simulink model "ofdm_14b"  (Simulink 8.5)
settings: Solver=FixedStepDiscrete  SolverMode=SingleTasking  StartTime=0.0  StopTime=inf  MaxStep=1/(100*40e6)  RelTol=1e-3
PreLoadFcn:
  | Fsymbol              = .5e6;         % Symbol rate
  | D=8;  % decimation / interpolation
  | Bits_per_Symbol = 2;
  | Fbit  = Bits_per_Symbol*Fsymbol;
  | 
  | FFT_Size  = 64;
  | Cyclic        = 16;
  | Pilots         = 16;
  | Pilot_Level = 8;
  | Zero_Pad  = 3;
  | QAM_Level = 6;
  | 
  | OFDM_Frame =  FFT_Size+Cyclic;
  | Symbols_per_Frame = FFT_Size-Pilots-Zero_Pad;
  | 
  | Bits_per_Frame = Bits_per_Symbol*Symbols_per_Frame;
  | 
  | F_nco = Fsymbol*D*OFDM_Frame/(Symbols_per_Frame);
  | nco_nominal=2/D;
  | 
  | 
  | Fdelay = 8;  % rrc filter delay
  | Alpha = .25;  % excess BW
  | %rrc_coef=rcosine(1,D,'fir/sqrt',Alpha,Fdelay);
  | %rrc_coef=rrc_coef/sum(rrc_coef);
  | 
  | DPS=fdesign.pulseshaping(D,'Square Root Raised Cosine','Nsym,Beta',2*Fdelay,Alpha);
  | Hd=design(DPS);
  | rrc_coef=Hd.Numerator;
  | % force DC gain to unity.
  | rrc_coef=rrc_coef/sum(rrc_coef);
  | 
  | % coefficents for Farrow filter
  | b3 = [1/6 -1/2  1/2 -1/6];
  | b2 = [1/2 -1    1/2  0];
  | b1 = [1/3  1/2 -1    1/6];
  | b0 = [0    1    0    0];
StartFcn:
  | tic
StopFcn:
  | trun=toc
undefined symbols (not defined in the file): dfilt, Fs, j, magnitude
libraries: simulink x16, dspobslib x5, dspxfrm3 x4, dspstat3 x4, dspsnks4 x3, commchan3 x2, commrandsrc2 x2, commdigbbndam3 x2, dspsrcs4 x2, dspbuff3 x2, dsppolyfun x1, commsink2 x1
(part 2 of 2)

== system ofdm_14b/OFDM Transmitter with Variable Symbol Timing and Carrier Frequency Error/OFDM Symbol Gen/OFDM Generator ==
  note: set data signal level
  in_data : Inport  OutDataTypeStr=uint8
  Enable : EnablePort
  Buffer : Buffer  N=Bits_per_Frame  TreatMby1Signals=One channel
  Frame Conversion : FrameConversion  OutFrame=Sample-based
  Gain : Gain  Gain=D
  Gain1 : Gain  Gain=QAM_Level  SaturateOnIntegerOverflow=on  OutDataTypeStr=Inherit: Same as input  ParamDataTypeStr=Inherit: Same as input
  OFDM Transmitter1 : Subsystem
      mask Display: disp('OFDM\nTransmitter')
  Rectangular QAM Modulator Baseband1 : commdigbbndam3/Rectangular QAM Modulator Baseband  M=4  InType=Bit  Enc=Binary  Mapping=[0:15]  PowType=Min. distance between symbols  MinDist=2  AvgPow=1  PeakPow=1  Ph=0  outDtype=Fixed-point  outWordLen=12  outUDDataType=sfix(16)  outFracLenMode=User-defined  outFracLen=7
  Out1 : Outport
  wires:
  Buffer/1 -> Rectangular QAM Modulator Baseband1/1
  OFDM Transmitter1/1(Out) -> Gain/1
  Rectangular QAM Modulator Baseband1/1 -> Gain1/1
  Gain/1 -> Frame Conversion/1
  Gain1/1 -> OFDM Transmitter1/1(In)
  Frame Conversion/1 -> Out1/1
  in_data/1 -> Buffer/1

== system ofdm_14b/OFDM Transmitter with Variable Symbol Timing and Carrier Frequency Error/Timing Control Unit1/S&H 1 ==
  In1 : Inport
  Enable : EnablePort
  Out1 : Outport
  wires:
  In1/1 -> Out1/1

== system ofdm_14b/OFDM Transmitter with Variable Symbol Timing and Carrier Frequency Error/Timing Control Unit1/Scaling1 ==
  note: This Division can be eliminated
      | and replaced by a mpy by constant
      | for small variations (< 1%)
      | about an operating point.
  In1 : Inport
  In2 : Inport  Port=2
  Add : Sum  Inputs=-+
  Constant : Constant
  Divide : Product  Inputs=*/
  Out1 : Outport
  wires:
  In2/1 -> Divide/2
  In1/1 -> Add/1
  Constant/1 -> Add/2
  Add/1 -> Divide/1
  Divide/1 -> Out1/1

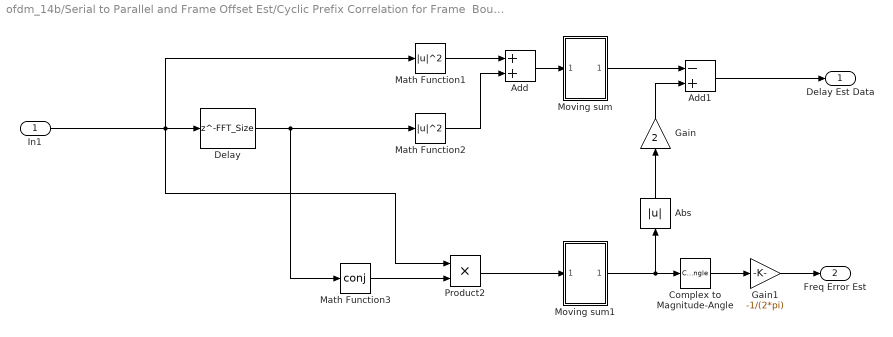
== system ofdm_14b/Serial to Parallel and Frame Offset Est/Cyclic Prefix Correlation for Frame  Boundary Estimation/Estimators ==
  In1 : Inport
  Abs : Abs
  Add : Sum
  Add1 : Sum  Inputs=-+
  Complex to Magnitude-Angle : ComplexToMagnitudeAngle  Output=Angle
  Delay : Delay  DelayLength=FFT_Size  InitialCondition=0
  Gain : Gain  Gain=2
  Gain1 : Gain  Gain=-1/(2*pi)
  Math Function1 : Math  Operator=magnitude^2  SaturateOnIntegerOverflow=on
  Math Function2 : Math  Operator=magnitude^2  SaturateOnIntegerOverflow=on
  Math Function3 : Math  Operator=conj  SaturateOnIntegerOverflow=on
  Moving sum : Subsystem
  Moving sum1 : Subsystem
  Product2 : Product  RndMeth=Zero
  Delay Est Data : Outport
  Freq Error Est : Outport  Port=2
  wires:
  In1/1 -> Product2/1, Delay/1, Math Function1/1
  Gain1/1 -> Freq Error Est/1
  Complex to Magnitude-Angle/1 -> Gain1/1
  Math Function3/1 -> Product2/2
  Gain/1 -> Add1/2
  Abs/1 -> Gain/1
  Add1/1 -> Delay Est Data/1
  Moving sum/1(Out1) -> Add1/1
  Moving sum1/1(Out1) -> Complex to Magnitude-Angle/1, Abs/1
  Product2/1 -> Moving sum1/1(In1)
  Add/1 -> Moving sum/1(In1)
  Math Function2/1 -> Add/2
  Math Function1/1 -> Add/1
  Delay/1 -> Math Function3/1, Math Function2/1

== system ofdm_14b/Serial to Parallel and Frame Offset Est/Cyclic Prefix Correlation for Frame  Boundary Estimation/Find max ==
  In1 : Inport
  Enable : EnablePort
  Add : Sum  Inputs=+-
  Constant : Constant  Value=OFDM_Frame/2
  Frame Conversion : FrameConversion  OutFrame=Sample-based
  Maximum : dspstat3/Maximum  fcn=Index  reset=None  InputProcessing=Columns as channels (frame based)  indexBase=One  operateOver=Each column  Dimension=1  colComp=on  operation=maximum  roiEnable=off  roiType=Rectangles  roiPortion=Entire ROI  roiOutput=Individual statistics for each ROI  roiFlag=off  accumDataTypeStr=Inherit: Same as product output  accumLastDataTypeStr=Inherit: Same as product output  roundingMode=Floor  overflowMode=off
  Moving sum : Subsystem
  reorder to center 0 point : Selector  InputPortWidth=80  Indices=[(OFDM_Frame/2+1):80 1:OFDM_Frame/2]
  Frame Offset Est : Outport  InitialOutput=0
  wires:
  In1/1 -> reorder to center 0 point/1
  Maximum/1 -> Frame Conversion/1
  reorder to center 0 point/1 -> Maximum/1
  Frame Conversion/1 -> Add/1
  Add/1 -> Moving sum/1(In1)
  Constant/1 -> Add/2
  Moving sum/1(Out1) -> Frame Offset Est/1

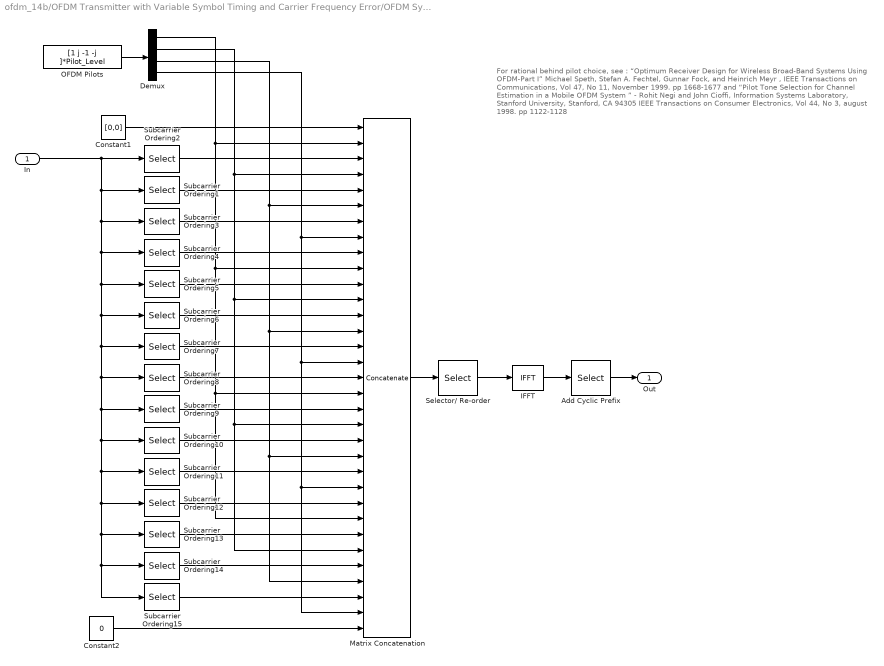
== system ofdm_14b/OFDM Transmitter with Variable Symbol Timing and Carrier Frequency Error/OFDM Symbol Gen/OFDM Generator/OFDM Transmitter1 ==
  note: For rational behind pilot choice, see :
      | “Optimum Receiver Design for Wireless Broad-Band Systems Using OFDM-Part I”
      | Michael Speth, Stefan A. Fechtel, Gunnar Fock, and Heinrich Meyr ,
      |  IEEE Transactions on Communications, Vol 47, No 11, November 1999. pp 1668-1677
      | and
      | “Pilot Tone Selection for Channel Estimation in a Mobile OFDM System ” -
      |  Rohit Negi and John Cioffi, Information Systems Laboratory, Stanford University, Stanford, CA 94305
      | IEEE Transactions on Consumer Electronics, Vol 44, No 3, august 1998. pp 1122-1128
  In : Inport
  Add Cyclic Prefix : Selector  InputPortWidth=64  Indices=[49:64 1:64]
  Constant1 : Constant  Value=[0,0]  OutDataTypeStr=fixdt(1,12,7)
  Constant2 : Constant  Value=0  OutDataTypeStr=fixdt(1,12,7)
  Demux : Demux
  IFFT : dspxfrm3/IFFT  CompMethod=Table lookup  TableOpt=HYBRID  TableOptActive=Speed  BitRevOrder=off  cs_in=off  SkipNorm=on  InheritFFTLength=on  FFTLength=64  WrapInput=on  mode=Complex  outSamplingMode=Frame based  RowConvenienceOn=on  FFTImplementation=Auto  firstCoeffDataTypeStr=Inherit: Same word length as input  firstCoeffLastDataTypeStr=Inherit: Same word length as input  outputMin=[]  outputMax=[]  roundingMode=Floor  overflowMode=off
  Matrix Concatenation : Concatenate  NumInputs=33  Mode=Multidimensional array
  OFDM Pilots : Constant  Value="[1 j -1 -j   ]*Pilot_Level"  OutDataTypeStr=fixdt(1,12,7)
  Selector/ Re-order : Selector  InputPortWidth=64  Indices=[33:64 1:32]
  Subcarrier Ordering1 : Selector  InputPortWidth=Symbols_per_Frame  Indices=4:6
  Subcarrier Ordering10 : Selector  InputPortWidth=Symbols_per_Frame  Indices=28:30
  Subcarrier Ordering11 : Selector  InputPortWidth=Symbols_per_Frame  Indices=31:33
  Subcarrier Ordering12 : Selector  InputPortWidth=Symbols_per_Frame  Indices=34:36
  Subcarrier Ordering13 : Selector  InputPortWidth=Symbols_per_Frame  Indices=37:39
  Subcarrier Ordering14 : Selector  InputPortWidth=Symbols_per_Frame  Indices=40:42
  Subcarrier Ordering15 : Selector  InputPortWidth=Symbols_per_Frame  Indices=43:45
  Subcarrier Ordering2 : Selector  InputPortWidth=Symbols_per_Frame  Indices=1:3
  Subcarrier Ordering3 : Selector  InputPortWidth=Symbols_per_Frame  Indices=7:9
  Subcarrier Ordering4 : Selector  InputPortWidth=Symbols_per_Frame  Indices=10:12
  Subcarrier Ordering5 : Selector  InputPortWidth=Symbols_per_Frame  Indices=13:15
  Subcarrier Ordering6 : Selector  InputPortWidth=Symbols_per_Frame  Indices=16:18
  Subcarrier Ordering7 : Selector  InputPortWidth=Symbols_per_Frame  Indices=19:21
  Subcarrier Ordering8 : Selector  InputPortWidth=Symbols_per_Frame  Indices=22:24
  Subcarrier Ordering9 : Selector  InputPortWidth=Symbols_per_Frame  Indices=25:27
  Out : Outport
  wires:
  In/1 -> Subcarrier Ordering14/1, Subcarrier Ordering15/1, Subcarrier Ordering13/1, Subcarrier Ordering12/1, Subcarrier Ordering11/1, Subcarrier Ordering10/1, Subcarrier Ordering9/1, Subcarrier Ordering8/1, Subcarrier Ordering7/1, Subcarrier Ordering6/1, Subcarrier Ordering5/1, Subcarrier Ordering4/1, Subcarrier Ordering3/1, Subcarrier Ordering1/1, Subcarrier Ordering2/1
  IFFT/1 -> Add Cyclic Prefix/1
  Matrix Concatenation/1 -> Selector/ Re-order/1
  Selector/ Re-order/1 -> IFFT/1
  Subcarrier Ordering2/1 -> Matrix Concatenation/3
  Subcarrier Ordering1/1 -> Matrix Concatenation/5
  Subcarrier Ordering3/1 -> Matrix Concatenation/7
  Subcarrier Ordering4/1 -> Matrix Concatenation/9
  Subcarrier Ordering5/1 -> Matrix Concatenation/11
  Subcarrier Ordering6/1 -> Matrix Concatenation/13
  Subcarrier Ordering7/1 -> Matrix Concatenation/15
  Subcarrier Ordering8/1 -> Matrix Concatenation/17
  Subcarrier Ordering9/1 -> Matrix Concatenation/19
  Subcarrier Ordering10/1 -> Matrix Concatenation/21
  Subcarrier Ordering11/1 -> Matrix Concatenation/23
  Subcarrier Ordering12/1 -> Matrix Concatenation/25
  Subcarrier Ordering13/1 -> Matrix Concatenation/27
  Subcarrier Ordering14/1 -> Matrix Concatenation/29
  Subcarrier Ordering15/1 -> Matrix Concatenation/31
  Add Cyclic Prefix/1 -> Out/1
  Constant1/1 -> Matrix Concatenation/1
  Constant2/1 -> Matrix Concatenation/33
  Demux/2 -> Matrix Concatenation/4, Matrix Concatenation/12, Matrix Concatenation/20, Matrix Concatenation/28
  Demux/3 -> Matrix Concatenation/6, Matrix Concatenation/14, Matrix Concatenation/22, Matrix Concatenation/30
  Demux/4 -> Matrix Concatenation/8, Matrix Concatenation/16, Matrix Concatenation/24, Matrix Concatenation/32
  OFDM Pilots/1 -> Demux/1
  Demux/1 -> Matrix Concatenation/26, Matrix Concatenation/18, Matrix Concatenation/10, Matrix Concatenation/2

== system ofdm_14b/Serial to Parallel and Frame Offset Est/Cyclic Prefix Correlation for Frame  Boundary Estimation/Estimators/Moving sum ==
  In1 : Inport
  Gain : Gain  Gain=1/Cyclic  SaturateOnIntegerOverflow=on  OutDataTypeStr=Inherit: Same as input  ParamDataTypeStr=Inherit: Same as input
  Integer Delay : Delay  DelayLength=Cyclic  InputProcessing=Inherited
  Integer Delay1 : Delay  DelayLength=1  InputProcessing=Inherited
  Sum2 : Sum  Inputs=|+-
  Sum3 : Sum  Inputs=|++
  Out1 : Outport
  wires:
  Gain/1 -> Out1/1
  In1/1 -> Sum2/1, Integer Delay/1
  Sum2/1 -> Sum3/1
  Integer Delay1/1 -> Sum3/2
  Sum3/1 -> Gain/1, Integer Delay1/1
  Integer Delay/1 -> Sum2/2

== system ofdm_14b/Serial to Parallel and Frame Offset Est/Cyclic Prefix Correlation for Frame  Boundary Estimation/Estimators/Moving sum1 ==
  In1 : Inport
  Gain : Gain  Gain=1/Cyclic  SaturateOnIntegerOverflow=on  OutDataTypeStr=Inherit: Same as input  ParamDataTypeStr=Inherit: Same as input
  Integer Delay : Delay  DelayLength=Cyclic  InputProcessing=Inherited
  Integer Delay1 : Delay  DelayLength=1  InputProcessing=Inherited
  Sum2 : Sum  Inputs=|+-
  Sum3 : Sum  Inputs=|++
  Out1 : Outport
  wires:
  Integer Delay/1 -> Sum2/2
  Sum3/1 -> Integer Delay1/1, Gain/1
  Integer Delay1/1 -> Sum3/2
  Sum2/1 -> Sum3/1
  In1/1 -> Integer Delay/1, Sum2/1
  Gain/1 -> Out1/1

== system ofdm_14b/Serial to Parallel and Frame Offset Est/Cyclic Prefix Correlation for Frame  Boundary Estimation/Find max/Moving sum ==
  In1 : Inport
  Gain : Gain  Gain=1/4  SaturateOnIntegerOverflow=on  OutDataTypeStr=Inherit: Same as input  ParamDataTypeStr=Inherit: Same as input
  Integer Delay : Delay  DelayLength=4  InputProcessing=Inherited
  Integer Delay1 : Delay  DelayLength=1  InitialCondition=0  InputProcessing=Inherited
  Sum2 : Sum  Inputs=|+-
  Sum3 : Sum  Inputs=|++
  Out1 : Outport
  wires:
  Integer Delay/1 -> Sum2/2
  Sum3/1 -> Integer Delay1/1, Gain/1
  Integer Delay1/1 -> Sum3/2
  Sum2/1 -> Sum3/1
  In1/1 -> Integer Delay/1, Sum2/1
  Gain/1 -> Out1/1
